simulink model "edsonSimulationv22"  (R2022b)
settings: Solver=VariableStepAuto  StartTime=0.0  StopTime=80  FixedStep=1e-4  RelTol=1e-3
values from neighbouring files (symbols this model uses):
  c1 = input(40)    [control_ABFTISMC.m]
  D = [13.9269190731477, 0.478984747386228, 13.9043475853434, 0.479066331803849 ... (first row only)    [Hinf.m]    (also in control_ABFTISMC.m = [input(19), input(20), input(21); dinamic.m = - [X_u + X_uu * abs(u),              0,                   0; linealization.m = - [coef.X_u + coef.X_uu * abs(u_sym),              0,       )
  gamma = [atan2(diff(y_smooth),diff(x_smooth)), atan2(diff(y_smooth(end-1:end)),diff(x_smooth(end-1:end)))]    [trajectory.m]
  h1 = input(50)    [control_ABFTISMC.m]
  h2 = input(51)    [control_ABFTISMC.m]
  h3 = input(53)    [control_ABFTISMC.m]
  I_z = input(12)    [dinamic.m]    (also in linealization.m = coef.I_z; simulationParameters.m = 204.1)
  lambda1 = input(57)    [control_ABFTISMC.m]
  lambda2 = input(52)    [control_ABFTISMC.m]
  M = [input(1), input(2), input(3) ... (first row only)    [control_ABFTISMC.m]    (also in dinamic.m = [m - X_u_dot,           0,                      0; hinfController.m = 1.5; linealization.m = [coef.m - X_u_dot,           0,                      0)
  m = input(6)    [dinamic.m]    (also in simulationParameters.m = 250)
  N_ncnd = input(29)    [dinamic.m]    (also in simulationParameters.m = -1.5777)
  N_r = input(18)    [dinamic.m]    (also in simulationParameters.m = -741.1947; trajectory_2.m = 8.68555609659)
  N_r_dot = input(13)    [dinamic.m]    (also in linealization.m = coef.N_r_dot; simulationParameters.m = -748.3102)
  N_rnc = input(27)    [dinamic.m]    (also in simulationParameters.m = -2.8549)
  N_rr = input(19)    [dinamic.m]    (also in simulationParameters.m = -262.7909)
  N_und = input(28)    [dinamic.m]    (also in simulationParameters.m = 2.7616)
  N_v_dot = input(11)    [dinamic.m]    (also in linealization.m = coef.N_v_dot; simulationParameters.m = -370.5973)
  N_vnc = input(26)    [dinamic.m]    (also in simulationParameters.m = -0.5382)
  p = input(47)    [control_ABFTISMC.m]
  phi1 = input(49)    [control_ABFTISMC.m]
  q = input(48)    [control_ABFTISMC.m]
  r_0 = eps    [linealization.m]    (also in simulationParameters.m = 0)
  u_0 = 2.0    (= 2)    [linealization.m]    (also in simulationParameters.m = 0)
  v_0 = eps    [linealization.m]    (also in simulationParameters.m = 0)
  x_0 = 0    [linealization.m]    (also in simulationParameters.m)
  x_g = input(10)    [dinamic.m]    (also in linealization.m = coef.x_g; simulationParameters.m = 0.08)
  X_ncnc = input(22)    [dinamic.m]    (also in simulationParameters.m = 1.0518)
  X_ndnd = input(23)    [dinamic.m]    (also in simulationParameters.m = 1.0518)
  X_rnd = input(21)    [dinamic.m]    (also in simulationParameters.m = 1.8411)
  X_u = input(14)    [dinamic.m]    (also in simulationParameters.m = -0.2912)
  X_u_dot = input(7)    [dinamic.m]    (also in linealization.m = coef.X_u_dot; simulationParameters.m = -2.4706)
  X_unc = input(20)    [dinamic.m]    (also in simulationParameters.m = -3.6822)
  X_uu = input(15)    [dinamic.m]    (also in simulationParameters.m = -27.6262)
  y_0 = 0    [linealization.m]    (also in simulationParameters.m)
  Y_r_dot = input(9)    [dinamic.m]    (also in linealization.m = coef.Y_r_dot; simulationParameters.m = -370.5973)
  Y_rnc = -0.5382    [simulationParameters.m]
  Y_v = input(16)    [dinamic.m]    (also in simulationParameters.m = -123.5324)
  Y_v_dot = input(8)    [dinamic.m]    (also in linealization.m = coef.Y_v_dot; simulationParameters.m = -247.0649)
  Y_vnc = input(24)    [dinamic.m]    (also in simulationParameters.m = -0.3588)
  Y_vv = input(17)    [dinamic.m]    (also in simulationParameters.m = -38.9275)
  yaw_0 = 0    [linealization.m]    (also in simulationParameters.m)
undefined symbols (not defined in the file or in its folder): Delta, mu, q1, q2, set_point
libraries: simulink x6, slpidlib x2
settings Model: Creator=b_ant  LastModifiedBy=b_ant
settings OptimizationCC: ReuseModelBlockBuffer=on
settings RTWCC: GPUComputeCapability=5.0
settings ConfigComp: CovBoundaryAbsTol=1.0e-5

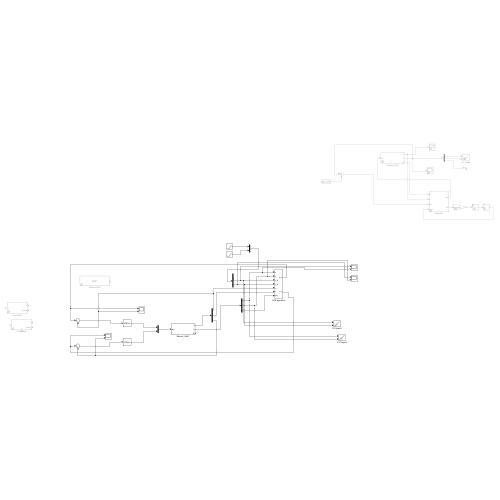
[thumbnail: Simulink's stored preview of the top-level diagram]
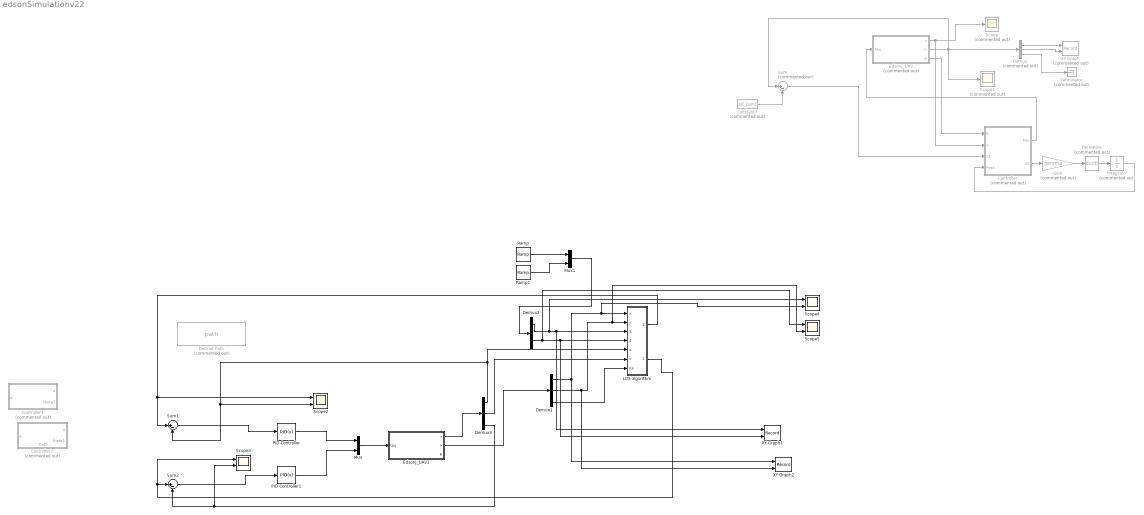
== system edsonSimulationv22 ==
  Constant3 : Constant  Commented=on  Value=set_point
  Controller : Subsystem  Commented=on
  Controller1 : Subsystem  Commented=on
  Controller2 : Subsystem  Commented=on
      settings: PortSchema="{\"entries\":[{\"content\":{\"sides\":[{\"content\":{\"connectorIds\":[\"In1\"]},\"type\":\"ConnectorPlacement.EquallySpacedRectSide\",\"uuid\":\"f76ee324-2c0a-46ef-be7a-d74aa6ee62a4\"},{\"content\":{\"connectorIds\":[\"Out1\",\"Out2\"],\"side\":\"RIGHT\"},\"type\":\"ConnectorPlacement.EquallySpacedRectSide\",\"uuid\":\"2ae83653-956d-4e34-a111-2446cf218777\"},{\"content\":{\"side\":\"TOP\"},\"type\":\"ConnectorPlacement.EquallySpacedRectSide\",\"uuid\":\"b0369baa-5e74-46b7-b4a5-7385998946b3\"},{\"content\":{\"connectorIds\":[\"Out3\"],\"side\":\"BOTTOM\"},\"type\":\"ConnectorPlacement.EquallySpacedRectSide\",\"uuid\":\"f37e4ee0-8a75-487e-ad57-80d8bf5ca30b\"}]},\"type\":\"ConnectorPlacement.EquallySpacedConnector\",\"uuid\":\"b2cb6c63-afa1-4294-a6da-6dcd429c1702\"}],\"packageUris\":[\"http://schema.mathworks.com/mf0/Connector/R2020b\"],\"version\":\"1.0\"}"
  Demux : Demux  Commented=on  Outputs=3
  Demux1 : Demux  Outputs=3
  Demux2 : Demux  Outputs=2
  Demux3 : Demux  Outputs=3
  Derivative : Derivative  Commented=on
  Desired Path : FromWorkspace  Commented=on  VariableName=path
  EdsonJ_UAV : Subsystem  Commented=on
  EdsonJ_UAV1 : Subsystem
  Gain : Gain  Commented=on  Gain=gamma
  Integrator : Integrator  Commented=on  InitialCondition=[0,0,0]'
  LOS algorithm : Subsystem
  Mux : Mux  Inputs=2
  Mux1 : Mux  Inputs=2
  PID Controller : slpidlib/PID Controller  Controller=PID  Form=Parallel  TimeDomain=Continuous-time  UseExternalTs=off  SampleTime=-1  IntegratorMethod=Forward Euler  FilterMethod=Forward Euler  ControllerParametersSource=internal  P=50000  I=100  UseKiTs=off  D=0  N=100  UseFilter=on  TunerSelectOption=Transfer Function Based (PID Tuner App)  InitialConditionSource=internal  InitialConditionForIntegrator=0  InitialConditionForFilter=0  DifferentiatorICPrevScaledInput=0  ExternalReset=none  TrackingMode=off  Kt=1  LimitOutput=off  SatLimitsSource=internal  UpperSaturationLimit=inf  LowerSaturationLimit=-inf  LinearizeAsGain=on  AntiWindupMode=none  Kb=1  LimitIntegrator=off  UpperIntegratorSaturationLimit=inf  LowerIntegratorSaturationLimit=-inf  POutMin=[]  POutMax=[]  IOutMin=[]  IOutMax=[]  DOutMin=[]  DOutMax=[]  NOutMin=[]  NOutMax=[]  SumOutMin=[]  SumOutMax=[]  SaturationOutMin=[]  SaturationOutMax=[]  PParamMin=[]  PParamMax=[]  IParamMin=[]  IParamMax=[]  DParamMin=[]  DParamMax=[]  NParamMin=[]  NParamMax=[]  KbParamMin=[]  KbParamMax=[]  KtParamMin=[]  KtParamMax=[]  KbOutMin=[]  KbOutMax=[]  KtOutMin=[]  KtOutMax=[]  IntegratorOutMin=[]  IntegratorOutMax=[]  FilterOutMin=[]  FilterOutMax=[]  SumI1OutMin=[]  SumI1OutMax=[]  SumI2OutMin=[]  SumI2OutMax=[]  SumI3OutMin=[]  SumI3OutMax=[]  SumI4OutMin=[]  SumI4OutMax=[]  SumDOutMin=[]  SumDOutMax=[]  DifferentiatorOutMin=[]  DifferentiatorOutMax=[]  FilterDiffOutCoefMin=[]  FilterDiffOutCoefMax=[]  ReciprocalOutMin=[]  ReciprocalOutMax=[]  SumDenOutMin=[]  SumDenOutMax=[]  SumNumOutMin=[]  SumNumOutMax=[]  DivideOutMin=[]  DivideOutMax=[]  UdiffTsProdOutMin=[]  UdiffTsProdOutMax=[]  NTsProdOutMin=[]  NTsProdOutMax=[]  UintegralTsProdOutMin=[]  UintegralTsProdOutMax=[]  UngainTsProdOutMin=[]  UngainTsProdOutMax=[]  IntegratorContinuousStateAttributes=''  IntegratorStateMustResolveToSignalObject=off  IntegratorRTWStateStorageClass=Auto  FilterContinuousStateAttributes=''  FilterStateMustResolveToSignalObject=off  FilterRTWStateStorageClass=Auto  ParallelPVariant=InternalParameters  IdealPVariant=Disabled  IVariant=InternalParameters  DVariant=InternalParameters  IntegratorVariant=Continuous  SatVariant=Disabled  AWVariant=Passthrough  PCopyVariant=Disabled  TRVariant=Disabled  FdbkBlocksVariant=Forward  IdealPFdbkVariant=Disabled  SatFdbkVariant=Disabled  DerivativeFilterVariant=ContFilter  NVariant=InternalParameters  NCopyVariant=Disabled  FilterICVariant=InternalICsFilter  IntegratorICVariant=InternalICs  ExternalResetVariant=Disabled  TRSumVariant=Passthrough  SumFdbkVariant=Disabled  SumVariant=Sum_PID  TsampFilterVariant=InternalTs  TsampNgainVariant=Passthrough  TsampIntegralVariant=Disabled_SignalSpec  ExternalSaturationOutDataTypeStr=Inherit: Same as second input
  PID Controller1 : slpidlib/PID Controller  Controller=PID  Form=Parallel  TimeDomain=Continuous-time  UseExternalTs=off  SampleTime=-1  IntegratorMethod=Forward Euler  FilterMethod=Forward Euler  ControllerParametersSource=internal  P=50000  I=1000  UseKiTs=off  D=0  N=100  UseFilter=on  TunerSelectOption=Transfer Function Based (PID Tuner App)  InitialConditionSource=internal  InitialConditionForIntegrator=0  InitialConditionForFilter=0  DifferentiatorICPrevScaledInput=0  ExternalReset=none  TrackingMode=off  Kt=1  LimitOutput=off  SatLimitsSource=internal  UpperSaturationLimit=inf  LowerSaturationLimit=-inf  LinearizeAsGain=on  AntiWindupMode=none  Kb=1  LimitIntegrator=off  UpperIntegratorSaturationLimit=inf  LowerIntegratorSaturationLimit=-inf  POutMin=[]  POutMax=[]  IOutMin=[]  IOutMax=[]  DOutMin=[]  DOutMax=[]  NOutMin=[]  NOutMax=[]  SumOutMin=[]  SumOutMax=[]  SaturationOutMin=[]  SaturationOutMax=[]  PParamMin=[]  PParamMax=[]  IParamMin=[]  IParamMax=[]  DParamMin=[]  DParamMax=[]  NParamMin=[]  NParamMax=[]  KbParamMin=[]  KbParamMax=[]  KtParamMin=[]  KtParamMax=[]  KbOutMin=[]  KbOutMax=[]  KtOutMin=[]  KtOutMax=[]  IntegratorOutMin=[]  IntegratorOutMax=[]  FilterOutMin=[]  FilterOutMax=[]  SumI1OutMin=[]  SumI1OutMax=[]  SumI2OutMin=[]  SumI2OutMax=[]  SumI3OutMin=[]  SumI3OutMax=[]  SumI4OutMin=[]  SumI4OutMax=[]  SumDOutMin=[]  SumDOutMax=[]  DifferentiatorOutMin=[]  DifferentiatorOutMax=[]  FilterDiffOutCoefMin=[]  FilterDiffOutCoefMax=[]  ReciprocalOutMin=[]  ReciprocalOutMax=[]  SumDenOutMin=[]  SumDenOutMax=[]  SumNumOutMin=[]  SumNumOutMax=[]  DivideOutMin=[]  DivideOutMax=[]  UdiffTsProdOutMin=[]  UdiffTsProdOutMax=[]  NTsProdOutMin=[]  NTsProdOutMax=[]  UintegralTsProdOutMin=[]  UintegralTsProdOutMax=[]  UngainTsProdOutMin=[]  UngainTsProdOutMax=[]  IntegratorContinuousStateAttributes=''  IntegratorStateMustResolveToSignalObject=off  IntegratorRTWStateStorageClass=Auto  FilterContinuousStateAttributes=''  FilterStateMustResolveToSignalObject=off  FilterRTWStateStorageClass=Auto  ParallelPVariant=InternalParameters  IdealPVariant=Disabled  IVariant=InternalParameters  DVariant=InternalParameters  IntegratorVariant=Continuous  SatVariant=Disabled  AWVariant=Passthrough  PCopyVariant=Disabled  TRVariant=Disabled  FdbkBlocksVariant=Forward  IdealPFdbkVariant=Disabled  SatFdbkVariant=Disabled  DerivativeFilterVariant=ContFilter  NVariant=InternalParameters  NCopyVariant=Disabled  FilterICVariant=InternalICsFilter  IntegratorICVariant=InternalICs  ExternalResetVariant=Disabled  TRSumVariant=Passthrough  SumFdbkVariant=Disabled  SumVariant=Sum_PID  TsampFilterVariant=InternalTs  TsampNgainVariant=Passthrough  TsampIntegralVariant=Disabled_SignalSpec  ExternalSaturationOutDataTypeStr=Inherit: Same as second input
  Ramp : simulink/Sources/Ramp  slope=1  start=0  InitialOutput=0
  Ramp1 : simulink/Sources/Ramp  slope=3  start=0  InitialOutput=0
  Scope : Scope  Commented=on
  Scope1 : Scope  Commented=on
  Scope{2..5} (4 alike) : Scope  NumInputPorts=2
  Sum : Sum  Commented=on  Inputs=|+-
  Sum1 : Sum  Inputs=|+-
  Sum2 : Sum  Inputs=|+-
  Terminator : Terminator  Commented=on
  XY Graph : Record  Commented=on  FileSettingsInternal="{\"entries\":[{\"content\":{\"excelSettings\":{\"content\":{},\"type\":\"Streamout.ExcelSettings\"},\"parquetSettings\":{\"content\":{},\"type\":\"Streamout.ParquetSettings\"}},\"type\":\"Streamout.FileSettingStorage\",\"uuid\":\"\"}],\"packageUris\":[\"http:\\/\\/schema.mathworks.com\\/mf0\\/streamout_blocks\\/R2020a\"],\"version\":\"1.0\"}"  Layout=[1 1]  SignalsInternal="{\"entries\":[{\"content\":{\"signals\":[{\"content\":{\"blockPath\":[],\"dimensions\":[1],\"domain\":\"\",\"lineColor\":\"#a2142f\",\"plots\":[ 1 ],\"port\":1,\"signalID\":1,\"signalName\":\"Demux:1\"},\"type\":\"RecordBlkView.Signal\",\"uuid\":\"\"},{\"content\":{\"blockPath\":[],\"dimensions\":[1],\"domain\":\"\",\"lineColor\":\"#139fff\",\"plots\":[ 1 ],\"port\":2,\"signalID\":2,\"signalName\":\"Demux:2\"},\"type\":\"RecordBlkView.Signal\",\"uuid\":\"\"}]},\"type\":\"RecordBlkView.InputSignals\",\"uuid\":\"\"}],\"packageUris\":[\"http:\\/\\/schema.mathworks.com\\/mf0\\/streamout_blocks\\/R2020a\"],\"version\":\"1.0\"}"  VisualizationBindings="{\"xyplotplugin\":{\"info\":[{\"series\":[{\"bindingParametersList\":[{\"parameter\":\"X-Axis\",\"signalID\":1,\"signalName\":\"Demux:1\"},{\"parameter\":\"Y-Axis\",\"signalID\":2,\"signalName\":\"Demux:2\"}],\"seriesID\":0}],\"subplotID\":1}]}}"  CompatibilityTag=XY
  XY Graph1 : Record  FileSettingsInternal="{\"entries\":[{\"content\":{\"excelSettings\":{\"content\":{},\"type\":\"Streamout.ExcelSettings\"},\"parquetSettings\":{\"content\":{},\"type\":\"Streamout.ParquetSettings\"}},\"type\":\"Streamout.FileSettingStorage\",\"uuid\":\"\"}],\"packageUris\":[\"http:\\/\\/schema.mathworks.com\\/mf0\\/streamout_blocks\\/R2020a\"],\"version\":\"1.0\"}"  Layout=[1 1]  SignalsInternal="{\"entries\":[{\"content\":{\"signals\":[{\"content\":{\"blockPath\":[],\"dimensions\":[1],\"domain\":\"\",\"lineColor\":\"#a2142f\",\"plots\":[ 1 ],\"port\":1,\"signalID\":1,\"signalName\":\"Demux2:1\"},\"type\":\"RecordBlkView.Signal\",\"uuid\":\"\"},{\"content\":{\"blockPath\":[],\"dimensions\":[1],\"domain\":\"\",\"lineColor\":\"#139fff\",\"plots\":[ 1 ],\"port\":2,\"signalID\":2,\"signalName\":\"Demux2:2\"},\"type\":\"RecordBlkView.Signal\",\"uuid\":\"\"}]},\"type\":\"RecordBlkView.InputSignals\",\"uuid\":\"\"}],\"packageUris\":[\"http:\\/\\/schema.mathworks.com\\/mf0\\/streamout_blocks\\/R2020a\"],\"version\":\"1.0\"}"  VisualizationBindings="{\"xyplotplugin\":{\"info\":[{\"series\":[{\"bindingParametersList\":[{\"parameter\":\"X-Axis\",\"signalID\":1,\"signalName\":\"Demux2:1\"},{\"parameter\":\"Y-Axis\",\"signalID\":2,\"signalName\":\"Demux2:2\"}],\"seriesID\":0}],\"subplotID\":1}]}}"  CompatibilityTag=XY
  XY Graph2 : Record  FileSettingsInternal="{\"entries\":[{\"content\":{\"excelSettings\":{\"content\":{},\"type\":\"Streamout.ExcelSettings\"},\"parquetSettings\":{\"content\":{},\"type\":\"Streamout.ParquetSettings\"}},\"type\":\"Streamout.FileSettingStorage\",\"uuid\":\"\"}],\"packageUris\":[\"http:\\/\\/schema.mathworks.com\\/mf0\\/streamout_blocks\\/R2020a\"],\"version\":\"1.0\"}"  Layout=[1 1]  SignalsInternal="{\"entries\":[{\"content\":{\"signals\":[{\"content\":{\"blockPath\":[],\"dimensions\":[1],\"domain\":\"\",\"lineColor\":\"#a2142f\",\"plots\":[ 1 ],\"port\":1,\"signalID\":1,\"signalName\":\"Demux1:1\"},\"type\":\"RecordBlkView.Signal\",\"uuid\":\"\"},{\"content\":{\"blockPath\":[],\"dimensions\":[1],\"domain\":\"\",\"lineColor\":\"#139fff\",\"plots\":[ 1 ],\"port\":2,\"signalID\":2,\"signalName\":\"Demux1:2\"},\"type\":\"RecordBlkView.Signal\",\"uuid\":\"\"}]},\"type\":\"RecordBlkView.InputSignals\",\"uuid\":\"\"}],\"packageUris\":[\"http:\\/\\/schema.mathworks.com\\/mf0\\/streamout_blocks\\/R2020a\"],\"version\":\"1.0\"}"  VisualizationBindings="{\"xyplotplugin\":{\"info\":[{\"series\":[{\"bindingParametersList\":[{\"parameter\":\"X-Axis\",\"signalID\":1,\"signalName\":\"Demux1:1\"},{\"parameter\":\"Y-Axis\",\"signalID\":2,\"signalName\":\"Demux1:2\"}],\"seriesID\":0}],\"subplotID\":1}]}}"  CompatibilityTag=XY
  wires:
  EdsonJ_UAV/1(v) -> Scope/1, Controller/2(v)
  Demux/1 -> XY Graph/1
  Demux/2 -> XY Graph/2
  EdsonJ_UAV/3(R) -> Controller/1(R)
  Constant3/1 -> Sum/2
  Sum/1 -> Controller/3(z1)
  Controller/1(tau) -> EdsonJ_UAV/1(tau)
  Controller/2(s2) -> Gain/1
  Gain/1 -> Derivative/1
  Derivative/1 -> Integrator/1
  Integrator/1 -> Controller/4(Fest)
  Demux/3 -> Terminator/1
  EdsonJ_UAV/2(n) -> Sum/1, Demux/1, Scope1/1
  Demux2/1 -> Scope4/1, XY Graph1/1, LOS algorithm/3(x_d)
  Demux2/2 -> Scope5/1, XY Graph1/2, LOS algorithm/4(y_d)
  Demux1/3 -> LOS algorithm/7(psi)
  EdsonJ_UAV1/2(n) -> Demux1/1
  Demux1/1 -> Scope4/2, LOS algorithm/1(x), XY Graph2/1
  Demux1/2 -> XY Graph2/2, Scope5/2, LOS algorithm/2(y)
  EdsonJ_UAV1/1(v) -> Demux3/1
  Demux3/1 -> Scope2/2, Sum1/2, LOS algorithm/5(u)
  Demux3/2 -> LOS algorithm/6(v)
  Mux/1 -> EdsonJ_UAV1/1(tau)
  Demux3/3 -> Scope3/2, Sum2/2
  Mux1/1 -> Demux2/1
  Ramp/1 -> Mux1/1
  Sum1/1 -> PID Controller/1
  PID Controller/1 -> Mux/1
  PID Controller1/1 -> Mux/2
  Sum2/1 -> PID Controller1/1
  LOS algorithm/1(u_d) -> Sum1/1, Scope2/1
  LOS algorithm/2(r_d) -> Scope3/1, Sum2/1
  Ramp1/1 -> Mux1/2

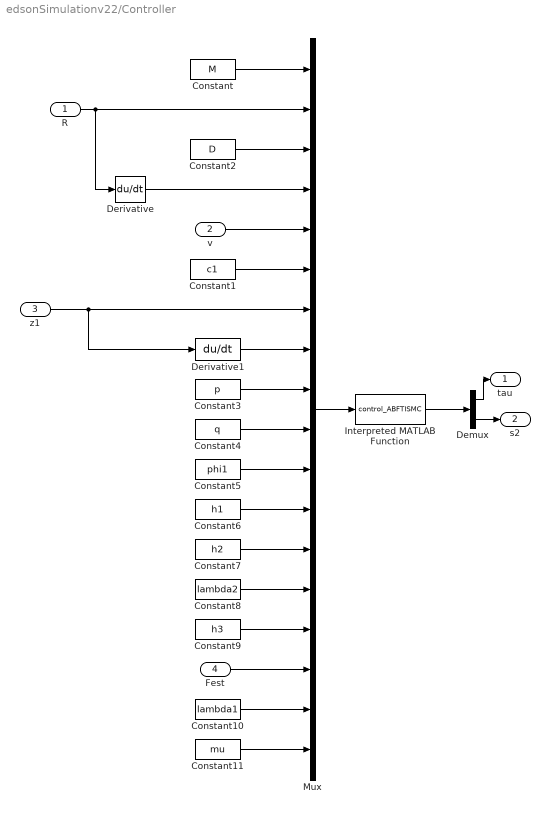
== system edsonSimulationv22/Controller ==
  R : Inport
  v : Inport  Port=2
  z1 : Inport  Port=3
  Fest : Inport  Port=4
  Constant : Constant  Value=M
  Constant1 : Constant  Value=c1
  Constant10 : Constant  Value=lambda1
  Constant11 : Constant  Value=mu
  Constant2 : Constant  Value=D
  Constant3 : Constant  Value=p
  Constant4 : Constant  Value=q
  Constant5 : Constant  Value=phi1
  Constant6 : Constant  Value=h1
  Constant7 : Constant  Value=h2
  Constant8 : Constant  Value=lambda2
  Constant9 : Constant  Value=h3
  Demux : Demux  Outputs=2
  Derivative : Derivative
  Derivative1 : Derivative
  Interpreted MATLAB Function : MATLABFcn  MATLABFcn=control_ABFTISMC
  Mux : Mux  Inputs=18
  tau : Outport
  s2 : Outport  Port=2
  wires:
  Mux/1 -> Interpreted MATLAB Function/1
  Constant/1 -> Mux/1
  R/1 -> Derivative/1, Mux/2
  Constant2/1 -> Mux/3
  Derivative/1 -> Mux/4
  v/1 -> Mux/5
  Constant1/1 -> Mux/6
  z1/1 -> Derivative1/1, Mux/7
  Derivative1/1 -> Mux/8
  Constant3/1 -> Mux/9
  Constant4/1 -> Mux/10
  Constant5/1 -> Mux/11
  Constant6/1 -> Mux/12
  Constant7/1 -> Mux/13
  Constant8/1 -> Mux/14
  Constant9/1 -> Mux/15
  Fest/1 -> Mux/16
  Interpreted MATLAB Function/1 -> Demux/1
  Demux/2 -> s2/1
  Demux/1 -> tau/1
  Constant10/1 -> Mux/17
  Constant11/1 -> Mux/18

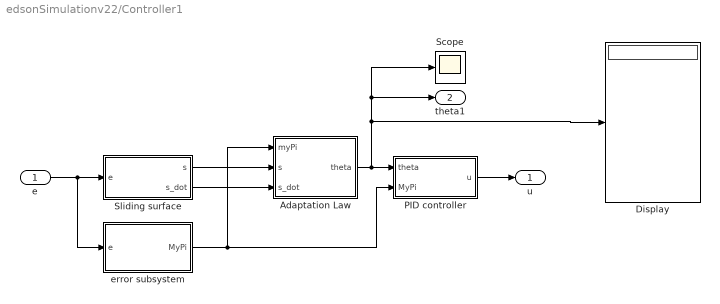
== system edsonSimulationv22/Controller1 ==
  e : Inport
  Adaptation Law : Subsystem  mask{alpha=q1.alpha, beta=q1.beta, epsilon=q1.epsilon, n=q1.n, kd0=q1.kd_init, ki0=q1.ki_init, kp0=q1.kp_init}
      mask prompts: kd0 "kd_0:"; ki0 "ki_0:"; kp0 "kp_0:"
      mask TypeOptions alpha: alpha/Value
      mask TypeOptions beta: beta/Value
      mask TypeOptions epsilon: epsilon/Value
      mask TypeOptions n: n/Value
      mask TypeOptions kd0: kd0/Value
      mask TypeOptions ki0: ki0/Value
      mask TypeOptions kp0: kp0/Value
  Display : Display
  PID controller : Subsystem
  Scope : Scope
  Sliding surface : Subsystem  mask{Gain=q1.lambda}
      mask prompts: Gain "Simulink:blkprm_prompts:GainGain"
      mask TypeOptions Gain: Gain/Gain
      mask DialogControl Gain Prompt: Gain:
  error subsystem : Subsystem
  u : Outport
  theta1 : Outport  Port=2
  wires:
  Sliding surface/1(s) -> Adaptation Law/2(s)
  Sliding surface/2(s_dot) -> Adaptation Law/3(s_dot)
  PID controller/1(u) -> u/1
  Adaptation Law/1(theta) -> theta1/1, Scope/1, Display/1, PID controller/1(theta)
  error subsystem/1(MyPi) -> PID controller/2(MyPi), Adaptation Law/1(myPi)
  e/1 -> error subsystem/1(e), Sliding surface/1(e)

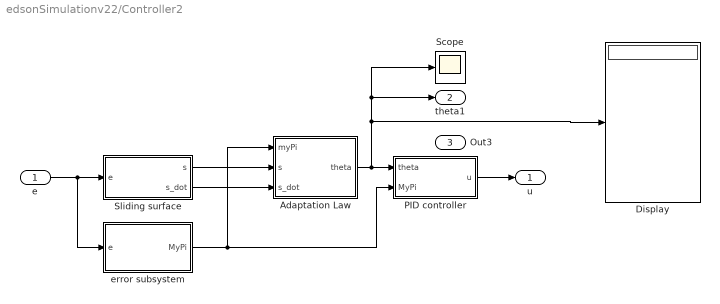
== system edsonSimulationv22/Controller2 ==
  e : Inport
  Adaptation Law : Subsystem  mask{alpha=q2.alpha, beta=q2.beta, epsilon=q2.epsilon, n=q2.n, kd0=q2.kd_init, ki0=q2.ki_init, kp0=q2.kp_init}
      mask prompts: kd0 "kd_0:"; ki0 "ki_0:"; kp0 "kp_0:"
      mask TypeOptions alpha: alpha/Value
      mask TypeOptions beta: beta/Value
      mask TypeOptions epsilon: epsilon/Value
      mask TypeOptions n: n/Value
      mask TypeOptions kd0: kd0/Value
      mask TypeOptions ki0: ki0/Value
      mask TypeOptions kp0: kp0/Value
  Display : Display
  PID controller : Subsystem
  Scope : Scope
  Sliding surface : Subsystem  mask{Gain=q2.lambda}
      mask prompts: Gain "Simulink:blkprm_prompts:GainGain"
      mask TypeOptions Gain: Gain/Gain
      mask DialogControl Gain Prompt: Gain:
  error subsystem : Subsystem
  u : Outport
  theta1 : Outport  Port=2
  Out3 : Outport  Port=3
  wires:
  Sliding surface/1(s) -> Adaptation Law/2(s)
  Sliding surface/2(s_dot) -> Adaptation Law/3(s_dot)
  PID controller/1(u) -> u/1
  Adaptation Law/1(theta) -> theta1/1, Scope/1, Display/1, PID controller/1(theta)
  error subsystem/1(MyPi) -> PID controller/2(MyPi), Adaptation Law/1(myPi)
  e/1 -> error subsystem/1(e), Sliding surface/1(e)

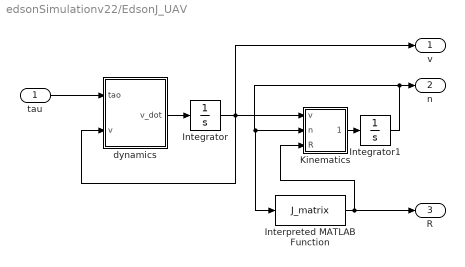
== system edsonSimulationv22/EdsonJ_UAV ==
  tau : Inport
  Integrator : Integrator  InitialCondition=[0,0,0]
  Integrator1 : Integrator  InitialCondition=[0,0,0]
  Interpreted MATLAB Function : MATLABFcn  MATLABFcn=J_matrix
  Kinematics : Subsystem
  dynamics : Subsystem
  v : Outport
  n : Outport  Port=2
  R : Outport  Port=3
  wires:
  Integrator/1 -> dynamics/2(v), v/1, Kinematics/1(v)
  dynamics/1(v_dot) -> Integrator/1
  Kinematics/1(n_dot) -> Integrator1/1
  Integrator1/1 -> n/1, Interpreted MATLAB Function/1, Kinematics/2(n)
  tau/1 -> dynamics/1(tao)
  Interpreted MATLAB Function/1 -> Kinematics/3(R), R/1

== system edsonSimulationv22/EdsonJ_UAV1 ==
  tau : Inport
  Interpreted MATLAB Function : MATLABFcn  MATLABFcn=J_matrix
  Kinematics : Subsystem
  dynamics : Subsystem
  v : Outport
  n : Outport  Port=2
  R : Outport  Port=3
  wires:
  dynamics/1(v_) -> Kinematics/1(v), dynamics/2(v), v/1
  Kinematics/1(n) -> n/1, Interpreted MATLAB Function/1
  tau/1 -> dynamics/1(tao)
  Interpreted MATLAB Function/1 -> R/1, Kinematics/2(J)

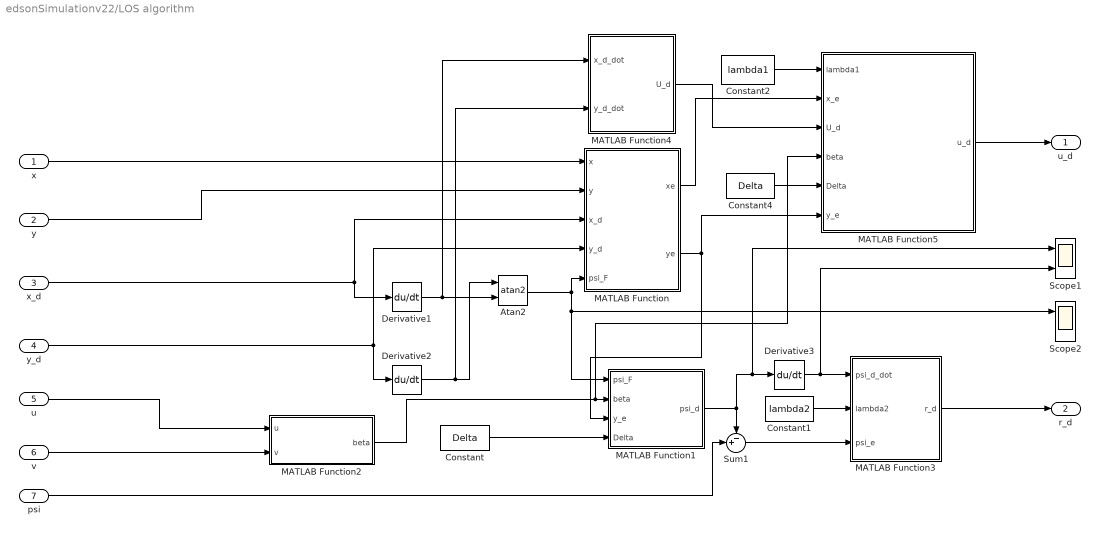
== system edsonSimulationv22/LOS algorithm ==
  x : Inport
  y : Inport  Port=2
  x_d : Inport  Port=3
  y_d : Inport  Port=4
  u : Inport  Port=5
  v : Inport  Port=6
  psi : Inport  Port=7
  Atan2 : Trigonometry  Operator=atan2
  Constant : Constant  Value=Delta
  Constant1 : Constant  Value=lambda2
  Constant2 : Constant  Value=lambda1
  Constant4 : Constant  Value=Delta
  Derivative1 : Derivative
  Derivative2 : Derivative
  Derivative3 : Derivative
  MATLAB Function : MATLAB Function  TreatAsAtomicUnit=on
  MATLAB Function1 : MATLAB Function  TreatAsAtomicUnit=on
  MATLAB Function2 : MATLAB Function  TreatAsAtomicUnit=on
  MATLAB Function3 : MATLAB Function  TreatAsAtomicUnit=on
  MATLAB Function4 : MATLAB Function  TreatAsAtomicUnit=on
  MATLAB Function5 : MATLAB Function  TreatAsAtomicUnit=on
  Scope1 : Scope  NumInputPorts=2
  Scope2 : Scope  NumInputPorts=2
  Sum1 : Sum  Inputs=-+|
  u_d : Outport
  r_d : Outport  Port=2
  wires:
  MATLAB Function1/1(psi_d) -> Scope1/1, Derivative3/1, Sum1/1
  MATLAB Function/2(ye) -> MATLAB Function1/3(y_e), MATLAB Function5/6(y_e)
  MATLAB Function2/1(beta) -> MATLAB Function5/4(beta), MATLAB Function1/2(beta)
  Derivative2/1 -> MATLAB Function4/2(y_d_dot), Atan2/1
  y_d/1 -> Derivative2/1, MATLAB Function/4(y_d)
  x_d/1 -> Derivative1/1, MATLAB Function/3(x_d)
  Constant/1 -> MATLAB Function1/4(Delta)
  MATLAB Function3/1(r_d) -> r_d/1
  y/1 -> MATLAB Function/2(y)
  Atan2/1 -> MATLAB Function/5(psi_F), MATLAB Function1/1(psi_F), Scope2/1
  Derivative1/1 -> MATLAB Function4/1(x_d_dot), Atan2/2
  MATLAB Function/1(xe) -> MATLAB Function5/2(x_e)
  Sum1/1 -> MATLAB Function3/3(psi_e)
  Derivative3/1 -> Scope1/2, MATLAB Function3/1(psi_d_dot)
  Constant1/1 -> MATLAB Function3/2(lambda2)
  Constant4/1 -> MATLAB Function5/5(Delta)
  Constant2/1 -> MATLAB Function5/1(lambda1)
  psi/1 -> Sum1/2
  MATLAB Function4/1(U_d) -> MATLAB Function5/3(U_d)
  x/1 -> MATLAB Function/1(x)
  MATLAB Function5/1(u_d) -> u_d/1
  v/1 -> MATLAB Function2/2(v)
  u/1 -> MATLAB Function2/1(u)

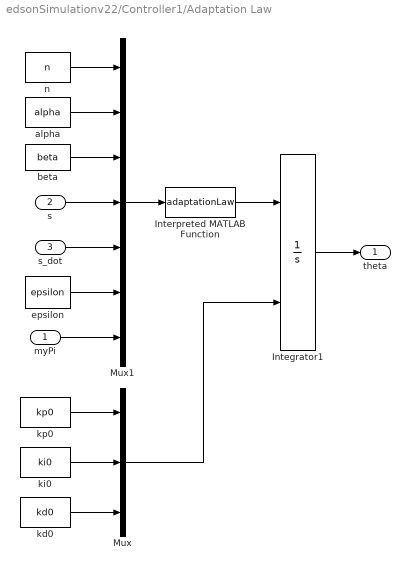
== system edsonSimulationv22/Controller1/Adaptation Law ==
  myPi : Inport
  s : Inport  Port=2
  s_dot : Inport  Port=3
  Integrator1 : Integrator  InitialConditionSource=external  InitialCondition=[1.460477259865257e-04,6.548069875818259e-05,0]
  Interpreted MATLAB Function : MATLABFcn  MATLABFcn=adaptationLaw
  Mux : Mux  Inputs=3
  Mux1 : Mux  Inputs=7
  alpha : Constant  Value=alpha
  beta : Constant  Value=beta
  epsilon : Constant  Value=epsilon
  kd0 : Constant  Value=kd0
  ki0 : Constant  Value=ki0
  kp0 : Constant  Value=kp0
  n : Constant  Value=n
  theta : Outport
  wires:
  alpha/1 -> Mux1/2
  Interpreted MATLAB Function/1 -> Integrator1/1
  myPi/1 -> Mux1/7
  s/1 -> Mux1/4
  epsilon/1 -> Mux1/6
  Integrator1/1 -> theta/1
  s_dot/1 -> Mux1/5
  beta/1 -> Mux1/3
  Mux1/1 -> Interpreted MATLAB Function/1
  n/1 -> Mux1/1
  ki0/1 -> Mux/2
  Mux/1 -> Integrator1/2
  kp0/1 -> Mux/1
  kd0/1 -> Mux/3

== system edsonSimulationv22/Controller1/PID controller ==
  theta : Inport
  MyPi : Inport  Port=2
  Interpreted MATLAB Function1 : MATLABFcn  MATLABFcn=controlLaw  OutputDimensions=1
  Mux2 : Mux  Inputs=2
  u : Outport
  wires:
  Mux2/1 -> Interpreted MATLAB Function1/1
  theta/1 -> Mux2/1
  Interpreted MATLAB Function1/1 -> u/1
  MyPi/1 -> Mux2/2

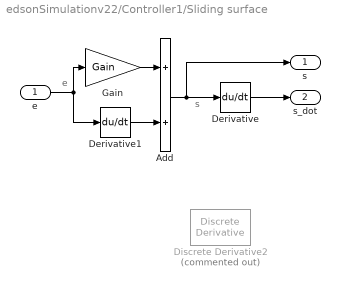
== system edsonSimulationv22/Controller1/Sliding surface ==
  note: s
  note: e
  e : Inport
  Add : Sum
  Derivative : Derivative
  Derivative1 : Derivative
  Discrete Derivative2 : simulink/Discrete/Discrete Derivative  Commented=on  gainval=1.0  ICPrevScaledInput=0.0  OutMin=[]  OutMax=[]  OutDataType=fixdt(1, 16)  OutScaling=2^-10  DoSatur=off
  Gain : Gain  Gain=Gain
  s : Outport
  s_dot : Outport  Port=2
  wires:
  Add/1 -> s/1, Derivative/1
  Gain/1 -> Add/1
  e/1 -> Derivative1/1, Gain/1
  Derivative1/1 -> Add/2
  Derivative/1 -> s_dot/1

== system edsonSimulationv22/Controller1/error subsystem ==
  e : Inport
  Derivative : Derivative
  Discrete Derivative1 : simulink/Discrete/Discrete Derivative  Commented=on  gainval=1.0  ICPrevScaledInput=0.0  OutMin=[]  OutMax=[]  OutDataType=fixdt(1, 16)  OutScaling=2^-10  DoSatur=off
  Integrator : Integrator
  Mux : Mux  Inputs=3
  MyPi : Outport
  wires:
  e/1 -> Derivative/1, Mux/1, Integrator/1
  Integrator/1 -> Mux/2
  Mux/1 -> MyPi/1
  Derivative/1 -> Mux/3

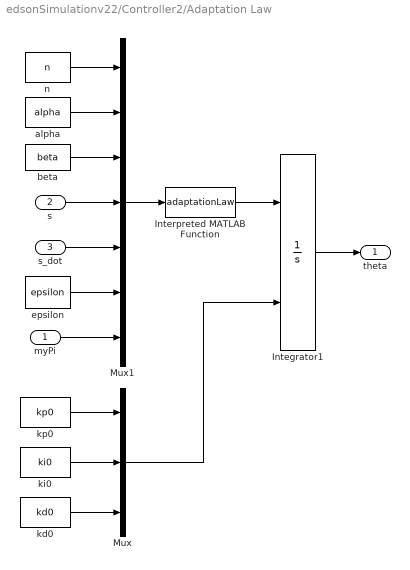
== system edsonSimulationv22/Controller2/Adaptation Law ==
  myPi : Inport
  s : Inport  Port=2
  s_dot : Inport  Port=3
  Integrator1 : Integrator  InitialConditionSource=external  InitialCondition=[1.460477259865257e-04,6.548069875818259e-05,0]
  Interpreted MATLAB Function : MATLABFcn  MATLABFcn=adaptationLaw
  Mux : Mux  Inputs=3
  Mux1 : Mux  Inputs=7
  alpha : Constant  Value=alpha
  beta : Constant  Value=beta
  epsilon : Constant  Value=epsilon
  kd0 : Constant  Value=kd0
  ki0 : Constant  Value=ki0
  kp0 : Constant  Value=kp0
  n : Constant  Value=n
  theta : Outport
  wires:
  alpha/1 -> Mux1/2
  Interpreted MATLAB Function/1 -> Integrator1/1
  myPi/1 -> Mux1/7
  s/1 -> Mux1/4
  epsilon/1 -> Mux1/6
  Integrator1/1 -> theta/1
  s_dot/1 -> Mux1/5
  beta/1 -> Mux1/3
  Mux1/1 -> Interpreted MATLAB Function/1
  n/1 -> Mux1/1
  ki0/1 -> Mux/2
  Mux/1 -> Integrator1/2
  kp0/1 -> Mux/1
  kd0/1 -> Mux/3

== system edsonSimulationv22/Controller2/PID controller ==
  theta : Inport
  MyPi : Inport  Port=2
  Interpreted MATLAB Function1 : MATLABFcn  MATLABFcn=controlLaw  OutputDimensions=1
  Mux2 : Mux  Inputs=2
  u : Outport
  wires:
  Mux2/1 -> Interpreted MATLAB Function1/1
  theta/1 -> Mux2/1
  Interpreted MATLAB Function1/1 -> u/1
  MyPi/1 -> Mux2/2

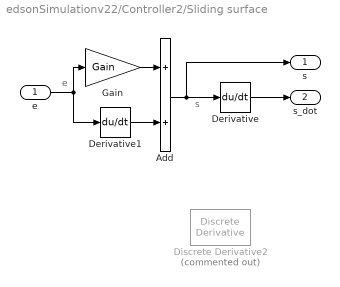
== system edsonSimulationv22/Controller2/Sliding surface ==
  note: s
  note: e
  e : Inport
  Add : Sum
  Derivative : Derivative
  Derivative1 : Derivative
  Discrete Derivative2 : simulink/Discrete/Discrete Derivative  Commented=on  gainval=1.0  ICPrevScaledInput=0.0  OutMin=[]  OutMax=[]  OutDataType=fixdt(1, 16)  OutScaling=2^-10  DoSatur=off
  Gain : Gain  Gain=Gain
  s : Outport
  s_dot : Outport  Port=2
  wires:
  Add/1 -> s/1, Derivative/1
  Gain/1 -> Add/1
  e/1 -> Derivative1/1, Gain/1
  Derivative1/1 -> Add/2
  Derivative/1 -> s_dot/1

== system edsonSimulationv22/Controller2/error subsystem ==
  e : Inport
  Derivative : Derivative
  Discrete Derivative1 : simulink/Discrete/Discrete Derivative  Commented=on  gainval=1.0  ICPrevScaledInput=0.0  OutMin=[]  OutMax=[]  OutDataType=fixdt(1, 16)  OutScaling=2^-10  DoSatur=off
  Integrator : Integrator
  Mux : Mux  Inputs=3
  MyPi : Outport
  wires:
  e/1 -> Derivative/1, Mux/1, Integrator/1
  Integrator/1 -> Mux/2
  Mux/1 -> MyPi/1
  Derivative/1 -> Mux/3

== system edsonSimulationv22/EdsonJ_UAV/Kinematics ==
  v : Inport
  n : Inport  Port=2
  R : Inport  Port=3
  Interpreted MATLAB Function1 : MATLABFcn  MATLABFcn=kinematic
  Mux : Mux  Inputs=3
  n_dot : Outport
  wires:
  n/1 -> Mux/2
  Mux/1 -> Interpreted MATLAB Function1/1
  v/1 -> Mux/1
  Interpreted MATLAB Function1/1 -> n_dot/1
  R/1 -> Mux/3

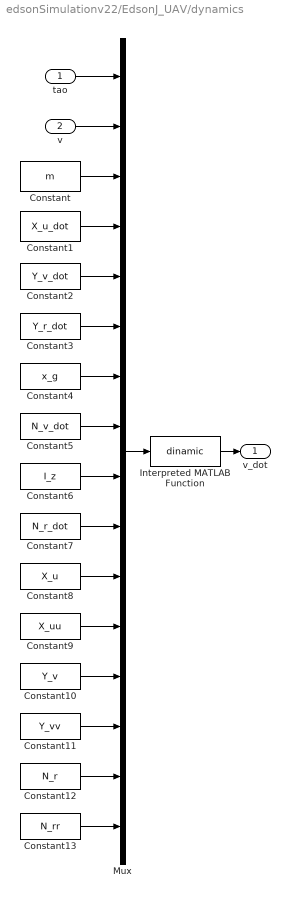
== system edsonSimulationv22/EdsonJ_UAV/dynamics ==
  tao : Inport
  v : Inport  Port=2
  Constant : Constant  Value=m
  Constant1 : Constant  Value=X_u_dot
  Constant10 : Constant  Value=Y_v
  Constant11 : Constant  Value=Y_vv
  Constant12 : Constant  Value=N_r
  Constant13 : Constant  Value=N_rr
  Constant2 : Constant  Value=Y_v_dot
  Constant3 : Constant  Value=Y_r_dot
  Constant4 : Constant  Value=x_g
  Constant5 : Constant  Value=N_v_dot
  Constant6 : Constant  Value=I_z
  Constant7 : Constant  Value=N_r_dot
  Constant8 : Constant  Value=X_u
  Constant9 : Constant  Value=X_uu
  Interpreted MATLAB Function : MATLABFcn  MATLABFcn=dinamic
  Mux : Mux  Inputs=16
  v_dot : Outport
  wires:
  tao/1 -> Mux/1
  Constant3/1 -> Mux/6
  Constant1/1 -> Mux/4
  Mux/1 -> Interpreted MATLAB Function/1
  v/1 -> Mux/2
  Constant/1 -> Mux/3
  Constant10/1 -> Mux/13
  Constant4/1 -> Mux/7
  Constant13/1 -> Mux/16
  Constant2/1 -> Mux/5
  Constant12/1 -> Mux/15
  Constant9/1 -> Mux/12
  Constant5/1 -> Mux/8
  Constant6/1 -> Mux/9
  Constant11/1 -> Mux/14
  Constant8/1 -> Mux/11
  Constant7/1 -> Mux/10
  Interpreted MATLAB Function/1 -> v_dot/1

== system edsonSimulationv22/EdsonJ_UAV1/Kinematics ==
  v : Inport
  J : Inport  Port=2
  Constant : Constant  Value=[x_0, y_0, yaw_0]
  Integrator1 : Integrator  InitialConditionSource=external  InitialCondition=[0,0,0]
  Interpreted MATLAB Function1 : MATLABFcn  MATLABFcn=kinematic
  Mux : Mux  Inputs=2
  n : Outport
  wires:
  Mux/1 -> Interpreted MATLAB Function1/1
  v/1 -> Mux/1
  J/1 -> Mux/2
  Interpreted MATLAB Function1/1 -> Integrator1/1
  Integrator1/1 -> n/1
  Constant/1 -> Integrator1/2

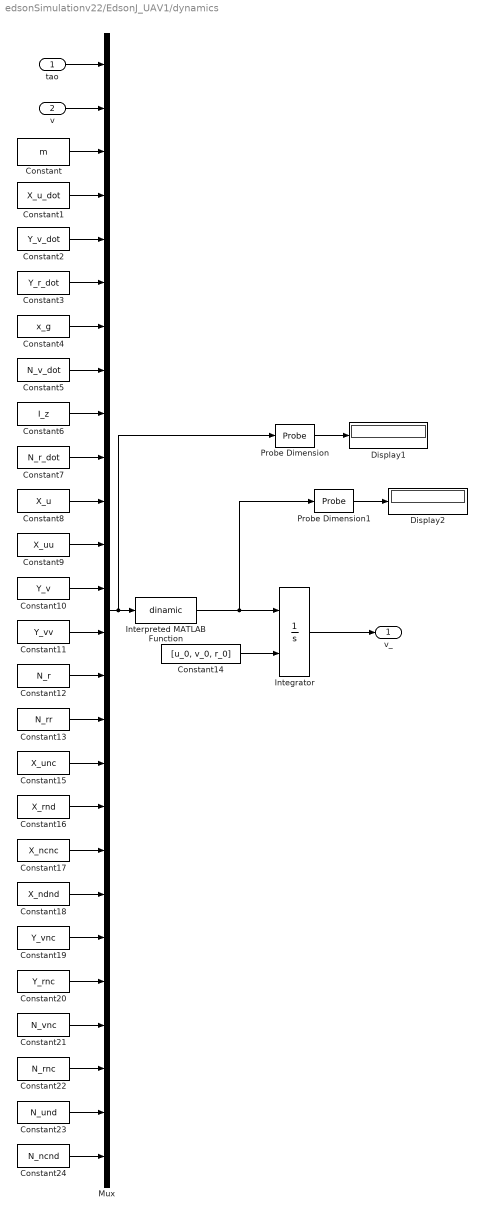
== system edsonSimulationv22/EdsonJ_UAV1/dynamics ==
  tao : Inport
  v : Inport  Port=2
  Constant : Constant  Value=m
  Constant1 : Constant  Value=X_u_dot
  Constant10 : Constant  Value=Y_v
  Constant11 : Constant  Value=Y_vv
  Constant12 : Constant  Value=N_r
  Constant13 : Constant  Value=N_rr
  Constant14 : Constant  Value=[u_0, v_0, r_0]
  Constant15 : Constant  Value=X_unc
  Constant16 : Constant  Value=X_rnd
  Constant17 : Constant  Value=X_ncnc
  Constant18 : Constant  Value=X_ndnd
  Constant19 : Constant  Value=Y_vnc
  Constant2 : Constant  Value=Y_v_dot
  Constant20 : Constant  Value=Y_rnc
  Constant21 : Constant  Value=N_vnc
  Constant22 : Constant  Value=N_rnc
  Constant23 : Constant  Value=N_und
  Constant24 : Constant  Value=N_ncnd
  Constant3 : Constant  Value=Y_r_dot
  Constant4 : Constant  Value=x_g
  Constant5 : Constant  Value=N_v_dot
  Constant6 : Constant  Value=I_z
  Constant7 : Constant  Value=N_r_dot
  Constant8 : Constant  Value=X_u
  Constant9 : Constant  Value=X_uu
  Display1 : Display
  Display2 : Display
  Integrator : Integrator  InitialConditionSource=external  InitialCondition=[0,0,0]
  Interpreted MATLAB Function : MATLABFcn  MATLABFcn=dinamic
  Mux : Mux  Inputs=26
  Probe Dimension : Probe  ProbeWidth=off  ProbeSampleTime=off  ProbeComplexSignal=off  ProbeSignalDimensions=on
  Probe Dimension1 : Probe  ProbeWidth=off  ProbeSampleTime=off  ProbeComplexSignal=off  ProbeSignalDimensions=on
  v_ : Outport
  wires:
  tao/1 -> Mux/1
  Constant3/1 -> Mux/6
  Constant1/1 -> Mux/4
  Mux/1 -> Probe Dimension/1, Interpreted MATLAB Function/1
  v/1 -> Mux/2
  Constant/1 -> Mux/3
  Constant10/1 -> Mux/13
  Constant4/1 -> Mux/7
  Constant13/1 -> Mux/16
  Constant2/1 -> Mux/5
  Constant12/1 -> Mux/15
  Constant9/1 -> Mux/12
  Constant5/1 -> Mux/8
  Constant6/1 -> Mux/9
  Constant11/1 -> Mux/14
  Constant8/1 -> Mux/11
  Constant7/1 -> Mux/10
  Integrator/1 -> v_/1
  Constant14/1 -> Integrator/2
  Constant15/1 -> Mux/17
  Constant16/1 -> Mux/18
  Constant17/1 -> Mux/19
  Constant18/1 -> Mux/20
  Constant19/1 -> Mux/21
  Constant20/1 -> Mux/22
  Constant21/1 -> Mux/23
  Constant22/1 -> Mux/24
  Constant23/1 -> Mux/25
  Constant24/1 -> Mux/26
  Probe Dimension/1 -> Display1/1
  Interpreted MATLAB Function/1 -> Probe Dimension1/1, Integrator/1
  Probe Dimension1/1 -> Display2/1

== matlab function edsonSimulationv22/LOS algorithm/MATLAB Function1 ==
  data: psi_F input; psi_d output; beta input; y_e input; Delta input
function psi_d = desired_yaw(psi_F, beta, y_e, Delta)
    psi_d = psi_F - beta + atan2(-y_e,Delta);
end

== matlab function edsonSimulationv22/LOS algorithm/MATLAB Function ==
  data: x input; xe output; y input; x_d input; y_d input; psi_F input; ye output
function [xe, ye] = error(x, y, x_d, y_d, psi_F)
%ERROR Computes the tracking error in the Frenet-Serret frame.
%
%   [xe, ye] = ERROR(x, y, x_d, y_d, psi_F) calculates the longitudinal (xe)
%   and lateral (ye) position error between the current position (x, y)
%   and the desired position (x_d, y_d), expressed in the Frenet-Serret frame.
%
%   Inputs:
%       x, y     - Current position coordinates
%       x_d, y_d - Desired position coordinates on the reference path
%       psi_F    - Heading angle (tangent direction) of the reference path at (x_d, y_d), in radians
%
%   Outputs:
%       xe - Longitudinal error (along the tangent direction)
%       ye - Lateral error (perpendicular to the path)

    % Rotation matrix from global to Frenet-Serret frame
    A = [ cos(psi_F), sin(psi_F);
         -sin(psi_F), cos(psi_F) ];

    % Position error in global coordinates
    pos_error = [x - x_d; y - y_d];

    % Transform error into Frenet-Serret frame
    local_error = A * pos_error;

    % Extract longitudinal and lateral components
    xe = local_error(1); % Tangential error
    ye = local_error(2); % Normal (lateral) error
end

== matlab function edsonSimulationv22/LOS algorithm/MATLAB Function2 ==
  data: u input; beta output; v input
function beta = beta_fun(u,v)
    beta = atan2(v,u);
end

== matlab function edsonSimulationv22/LOS algorithm/MATLAB Function3 ==
  data: r_d output; psi_d_dot input; lambda2 input; psi_e input
function r_d =  desired_yaw_rate(psi_d_dot, lambda2, psi_e)
    r_d = psi_d_dot - lambda2*psi_e;
end

== matlab function edsonSimulationv22/LOS algorithm/MATLAB Function4 ==
  data: x_d_dot input; U_d output; y_d_dot input
function U_d = desired_vel(x_d_dot, y_d_dot)
    U_d = (x_d_dot^2+y_d_dot^2)^(1/2);
end

== matlab function edsonSimulationv22/LOS algorithm/MATLAB Function5 ==
  data: lambda1 input; u_d output; x_e input; U_d input; beta input; Delta input; y_e input
function u_d = calcular_ud_LuoCheng(lambda1, x_e, U_d, beta, Delta, y_e)
termino_control = -lambda1 * x_e + U_d;

factor_geometrico_y_deriva = cos(beta) * (sqrt(Delta^2 + y_e^2) / Delta);

u_d = termino_control * factor_geometrico_y_deriva;
end
